simulink model "RCCar"  (R2016b)
settings: Solver=FixedStepAuto  StartTime=0.0  StopTime=10.0  RelTol=1e-3
undefined symbols (not defined in the file): AngleFactor, SpeedFactorFromMyTuning, SpeedfactorFromWeight
settings Model: Creator=NEATdemo  LastModifiedBy=NEATdemo

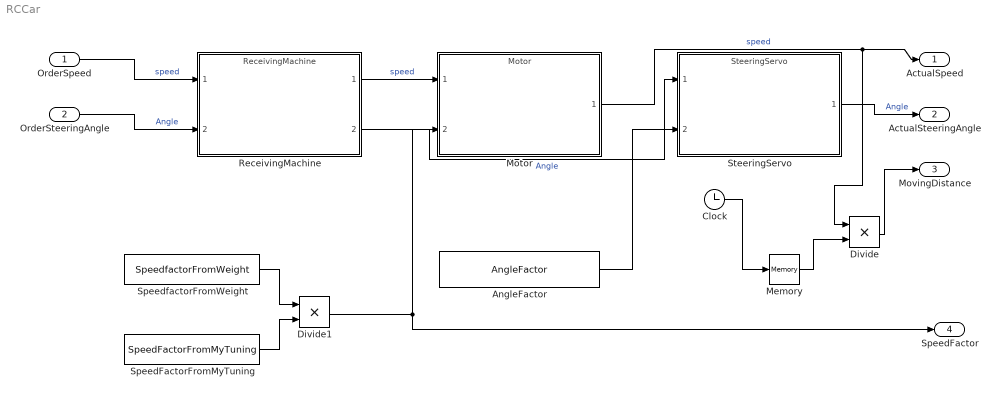
== system RCCar ==
  OrderSpeed : Inport
      settings: AttributesFormatString=speed
  OrderSteeringAngle : Inport  Port=2
      settings: AttributesFormatString=Angle
  AngleFactor : Constant  Value=AngleFactor
  Clock : Clock
  Divide : Product  Inputs=**
  Divide1 : Product  Inputs=**
  Memory : Memory
  Motor : ModelReference  ModelNameDialog=Motor  SimulationMode=Normal  ModelReferenceVersion=1.5
  ReceivingMachine : ModelReference  ModelNameDialog=ReceivingMachine  SimulationMode=Normal  ModelReferenceVersion=1.5
  SpeedFactorFromMyTuning : Constant  Value=SpeedFactorFromMyTuning
  SpeedfactorFromWeight : Constant  Value=SpeedfactorFromWeight
  SteeringServo : ModelReference  ModelNameDialog=SteeringServo  SimulationMode=Normal  ModelReferenceVersion=1.5
  ActualSpeed : Outport
      settings: AttributesFormatString=speed
  ActualSteeringAngle : Outport  Port=2
      settings: AttributesFormatString=Angle
  MovingDistance : Outport  Port=3
      settings: AttributesFormatString=Distance
  SpeedFactor : Outport  Port=4
      settings: AttributesFormatString=Distance
  wires:
  ReceivingMachine/1 -> Motor/1  "speed"
  ReceivingMachine/2 -> SteeringServo/1  "Angle"
  OrderSpeed/1 -> ReceivingMachine/1  "speed"
  OrderSteeringAngle/1 -> ReceivingMachine/2  "Angle"
  Motor/1 -> Divide/1, ActualSpeed/1  "speed"
  SteeringServo/1 -> ActualSteeringAngle/1  "Angle"
  Divide1/1 -> SpeedFactor/1, Motor/2
  AngleFactor/1 -> SteeringServo/2
  Memory/1 -> Divide/2
  Divide/1 -> MovingDistance/1
  Clock/1 -> Memory/1
  SpeedfactorFromWeight/1 -> Divide1/1
  SpeedFactorFromMyTuning/1 -> Divide1/2
